simulink model "SmallScaleMicroGrid"  (R2024a)
settings: Solver=ode23tb  StartTime=0  StopTime=60*60*24  FixedStep=1/(1000)  MaxStep=50  RelTol=1e-4
PreLoadFcn:
  | load('SmallScaleMicroGridSolarLoadData24h.mat')
values from neighbouring files (symbols this model uses):
  HPD_1min = [1086.95652174 1079.71014493 1072.46376812 1065.2173913 1057.97101449 1050.72463768 1043.47826087 1036.23188406 1028.98550725 1021.73913043 1014.49275362 1007.24637681 ... (1441 elements, 1441x1)]    [SmallScaleMicroGridSolarLoadData24h.mat]
  HPT_1min = [0 60 120 180 240 300 360 420 480 540 600 660 ... (1441 elements, 1441x1)]    [SmallScaleMicroGridSolarLoadData24h.mat]
  SPD_1min = [0 0 0 0 0 0 0 0 0 0 0 0 ... (1441 elements, 1441x1)]    [SmallScaleMicroGridSolarLoadData24h.mat]
  SPT_1min = [0 60 120 180 240 300 360 420 480 540 600 660 ... (1441 elements, 1441x1)]    [SmallScaleMicroGridSolarLoadData24h.mat]
libraries: spsCurrentMeasurementLib x4, spsControlledCurrentSourceLib x3, spsSeriesRLCBranchLib x3, spsACVoltageSourceLib x1, spsGroundLib x1, spsVoltageMeasurementLib x1, spspowerguiLib x1
settings Model: ModifiedByFormat=SPS  Creator=The MathWorks, Inc.  LastModifiedBy=SPS
settings SolverCC: InitialStep=1e-4  ZeroCrossAlgorithm=Adaptive  AlgebraicLoopSolver=TrustRegion  SolverResetMethod=Robust
settings DataIOCC: SaveFormat=Array  SaveOutput=off  SaveTime=off  ReturnWorkspaceOutputs=off  SignalLoggingName=sigsOut
settings OptimizationCC: BooleanDataType=off  ExpressionDepthLimit=2147483647  InitFltsAndDblsToZero=on  LifeSpan=inf
settings DebuggingCC: AlgebraicLoopMsg=none  SaveWithParameterizedLinksMsg=none  UnderspecifiedInitializationDetection=Classic  MergeDetectMultiDrivingBlocksExec=none  SignalResolutionControl=TryResolveAllWithWarning  MultiTaskDSMMsg=warning  MultiTaskCondExecSysMsg=none  FcnCallInpInsideContextMsg=warning  UnconnectedInputMsg=warning  UnconnectedOutputMsg=warning  UnconnectedLineMsg=warning  AllowSymbolicDim=off  StateNameClashWarn=warning  SubsystemReferenceDiagnosticForUnitTest=warning  SFUnexpectedBacktrackingDiag=warning  SFNoUnconditionalDefaultTransitionDiag=warning  SFExecutionAtInitializationDiag=none  ArithmeticOperatorsInVariantConditions=warning
settings HardwareCC: ProdBitPerPointer=32  ProdBitPerSizeT=32  ProdBitPerPtrDiffT=32  ProdLargestAtomicFloat=None  ProdIntDivRoundTo=Undefined  ProdEndianess=Unspecified  ProdWordSize=32  ProdHWDeviceType=32-bit Generic  TargetUnknown=on
settings ModelReferenceCC: EnableRefExpFcnMdlSchedulingChecks=on  PropagateSignalLabelsOutOfModel=off
settings SFSimCC: SimUseLocalCustomCode=off  CustomCodeUndefinedFunction=UseInterfaceOnly
settings RTWCC: RTWUseLocalCustomCode=off  GPUComputeCapability=3.5  DLArmComputeVersion=19.05
settings CodeAppCC: StateflowObjectComments=on
settings GRTTargetCC: TargetFcnLib=ansi_tfl_tmw.mat  TargetLangStandard=C89/C90 (ANSI)  CombineOutputUpdateFcns=off  GRTInterface=on
settings ConfigComp: CovMetricSettings=dw  CovSaveCumulativeToWorkspaceVar=on  CovSaveSingleToWorkspaceVar=on  CovExternalEMLEnable=off  CovSFcnEnable=off
settings SimscapeCC: SimscapeNormalizeSystem=off

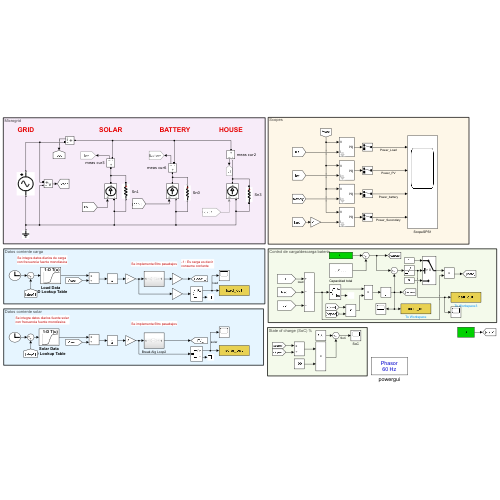
[thumbnail: Simulink's stored preview of the top-level diagram]
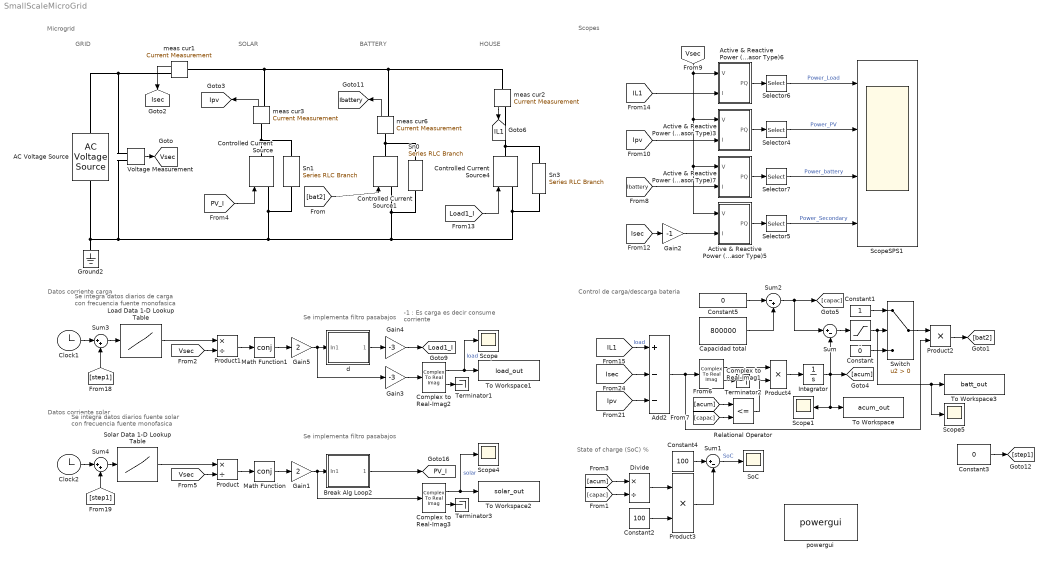
== system SmallScaleMicroGrid ==
  note: State of charge (SoC) %
  note: Control de carga/descarga bateria
  note: Microgrid
  note: Datos corriente solar
  note: Datos corriente carga
  note: SOLAR
  note: BATTERY
  note: HOUSE
  note: Se implementa filtro pasabajos
  note: Se integra datos diarios fuente solar
      | con frecuencia fuente monofasica
  note: Se integra datos diarios de carga
      | con frecuencia fuente monofasica
  note: Se implementa filtro pasabajos
  note: -1 : Es carga es decir
      | consume corriente
  note: GRID
  note: Scopes
  - : Saturate  UpperLimit=inf  LowerLimit=0
  AC Voltage Source : spsACVoltageSourceLib/AC Voltage Source  Amplitude=285  Phase=0  Frequency=60  SampleTime=0  Measurements=None  BusType=swing  Pref=10e3  Qref=0  Qmin=-inf  Qmax=+inf
  Active & Reactive Power (Phasor Type)3 : Subsystem  DialogController=POWERSYS.PowerSysDialog  mask(Active & Reactive Power (Phasor Type)){}
      mask help: Active & Reactive Power (Phasor Type)
      mask init:
      | power_initmask();
      mask Help: This block is part of a subset of blocks in the Extras library that does not have documentation associated with it, other than the block mask description.
      mask Display: disp('')
  Active & Reactive Power (Phasor Type)5 : Subsystem  DialogController=POWERSYS.PowerSysDialog  mask(Active & Reactive Power (Phasor Type)){}
      mask help: Active & Reactive Power (Phasor Type)
      mask init:
      | power_initmask();
      mask Help: This block is part of a subset of blocks in the Extras library that does not have documentation associated with it, other than the block mask description.
      mask Display: disp('')
  Active & Reactive Power (Phasor Type)6 : Subsystem  DialogController=POWERSYS.PowerSysDialog  mask(Active & Reactive Power (Phasor Type)){}
      mask help: Active & Reactive Power (Phasor Type)
      mask init:
      | power_initmask();
      mask Help: This block is part of a subset of blocks in the Extras library that does not have documentation associated with it, other than the block mask description.
      mask Display: disp('')
  Active & Reactive Power (Phasor Type)7 : Subsystem  DialogController=POWERSYS.PowerSysDialog  mask(Active & Reactive Power (Phasor Type)){}
      mask help: Active & Reactive Power (Phasor Type)
      mask init:
      | power_initmask();
      mask Help: This block is part of a subset of blocks in the Extras library that does not have documentation associated with it, other than the block mask description.
      mask Display: disp('')
  Add2 : Sum  Inputs=+--
  Break Alg Loop2 : Subsystem
  Capacidad total : Constant  Value=800000
  Clock1 : Clock
  Clock2 : Clock
  Complex to Real-Imag1 : ComplexToRealImag
  Complex to Real-Imag2 : ComplexToRealImag
  Complex to Real-Imag3 : ComplexToRealImag
  Constant : Constant  Value=0
  Constant1 : Constant
  Constant2 : Constant  Value=100
  Constant3 : Constant  Value=0
  Constant4 : Constant  Value=100
  Constant5 : Constant  Value=0
  Controlled Current Source : spsControlledCurrentSourceLib/Controlled Current Source  Initialize=on  Source_Type=AC  Amplitude=0  Phase=30  Frequency=60  Measurements=None
  Controlled Current Source1 : spsControlledCurrentSourceLib/Controlled Current Source  Initialize=on  Source_Type=AC  Amplitude=0  Phase=30  Frequency=60  Measurements=None
  Controlled Current Source4 : spsControlledCurrentSourceLib/Controlled Current Source  Initialize=on  Source_Type=AC  Amplitude=0  Phase=30  Frequency=60  Measurements=None
  Divide : Product  Inputs=*/
  Gain1 : Gain  Gain=2
  Gain2 : Gain  Gain=-1
  Gain3 : Gain  Gain=-3
  Gain4 : Gain  Gain=-3
  Gain5 : Gain  Gain=2
  Ground2 : spsGroundLib/Ground  LConnTagsString=a
  Integrator : Integrator
  Load Data 1-D Lookup Table : Lookup_n-D  NumberOfTableDimensions=1  BreakpointsForDimension1=HPT_1min  BeginIndexSearchUsingPreviousIndexResult=on  Table=HPD_1min  InternalRulePriority=Speed  RndMeth=Simplest
  Math Function : Math  Operator=conj
  Math Function1 : Math  Operator=conj
  Product : Product  Inputs=*/
  Product1 : Product  Inputs=*/
  Product2 : Product
  Product3 : Product
  Product4 : Product
  Relational Operator : RelationalOperator  Operator=<=  OutDataTypeStr=boolean  RndMeth=Simplest  InputSameDT=off
  Scope{,1,4..5} (4 alike) : Scope
  ScopeSPS1 : Scope  NumInputPorts=4
  Selector{4..7} (4 alike) : Selector  InputPortWidth=2  IndexOptions=Index vector (dialog)  Indices=1  OutputSizes=1
  Sn0 : spsSeriesRLCBranchLib/Series RLC Branch  LConnTagsString=__new0  RConnTagsString=__new0  BranchType=R  Resistance=1e6  Inductance=1e-3  SetiL0=off  InitialCurrent=0  Capacitance=1e-6  Setx0=off  InitialVoltage=0  Measurements=None
  Sn1 : spsSeriesRLCBranchLib/Series RLC Branch  LConnTagsString=__new0  RConnTagsString=__new0  BranchType=R  Resistance=1e6  Inductance=1e-3  SetiL0=off  InitialCurrent=0  Capacitance=1e-6  Setx0=off  InitialVoltage=0  Measurements=None
  Sn3 : spsSeriesRLCBranchLib/Series RLC Branch  LConnTagsString=__new0  RConnTagsString=__new0  BranchType=R  Resistance=1e6  Inductance=1e-3  SetiL0=off  InitialCurrent=0  Capacitance=1e-6  Setx0=off  InitialVoltage=0  Measurements=None
  SoC : Scope
  Solar Data 1-D Lookup Table : Lookup_n-D  NumberOfTableDimensions=1  BreakpointsForDimension1=SPT_1min  BeginIndexSearchUsingPreviousIndexResult=on  Table=SPD_1min  InternalRulePriority=Speed  RndMeth=Simplest
  Sum : Sum  Inputs=|+-
  Sum1 : Sum  Inputs=|+-
  Sum2 : Sum  Inputs=|-+
  Sum3 : Sum  Inputs=|++
  Sum4 : Sum  Inputs=|++
  Switch : Switch  Criteria=u2 > Threshold  SaturateOnIntegerOverflow=off  InputSameDT=off
  Terminator1 : Terminator
  Terminator2 : Terminator
  Terminator3 : Terminator
  To Workspace : ToWorkspace  VariableName=acum_out  SampleTime=-1
  To Workspace1 : ToWorkspace  VariableName=load_out  SampleTime=-1
  To Workspace2 : ToWorkspace  VariableName=solar_out  SampleTime=-1
  To Workspace3 : ToWorkspace  VariableName=batt_out  SampleTime=-1
  Voltage Measurement : spsVoltageMeasurementLib/Voltage Measurement  PhasorSimulation=on  OutputType=Complex  PSBequivalent=0
  d : Subsystem
  meas cur{1..3,6} (4 alike) : spsCurrentMeasurementLib/Current Measurement  PhasorSimulation=on  OutputType=Complex  PSBequivalent=0
  powergui : spspowerguiLib/powergui  SimulationMode=Phasor  SampleTime=1/60/100  frequency=60  Iterations=50  frequencyindice=60  Pbase=100e6  ErrMax=1e-4  UnitsV=kV  UnitsW=MW  buscounter=0  FunctionMessages=off  echomessages=off  EnableUseOfTLC=off  CurrentSourceSwitches=off  DisableSnubberDevices=off  DisableRonSwitches=off  DisableVfSwitches=off  DisplayEquations=off  AutomaticDiscreteSolvers=off  SolverType=Tustin  Interpol=off  ExternalGateDelay=off  methode=off  Ts=0  x0status=blocks  SPID=off  SwTol=0  HookPort=off  NonlinearTolerance=0  nMaxIteration=15  ContinueOnMaxIteration=off  RestoreLinks=warning  ResistiveCurrentMeasurement=off  Frange=[0:2:500]  Ylog=off  Xlog=on  ShowGrid=off  save=off  variable=ZData  structure=0  ZoomFFT=on  StartTime=0.0  cycles=1  DisplayStyle=1  fundamental=60  FreqAxis=off  MaxFrequency=1000  frequencyindicesteady=1  RmsSteady=1  display=off
  tag scope: IL1=global, Ibattery=global, Ipv=global, Isec=global, Load1_I=global, PV_I=global, Vsec=global
  wires:
  meas cur2/1 -> [IL1]
  meas cur1/1 -> [Isec]
  meas cur3/1 -> [Ipv]
  meas cur6/1 -> [Ibattery]
  Break Alg Loop2/1("1 ") -> [PV_I]
  Gain4/1 -> [Load1_I]
  Voltage Measurement/1 -> [Vsec]
  [Load1_I] -> Controlled Current Source4/1
  [PV_I] -> Controlled Current Source/1
  Load Data 1-D Lookup Table/1 -> Product1/1
  Product1/1 -> Math Function1/1
  Product/1 -> Math Function/1
  Solar Data 1-D Lookup Table/1 -> Product/1
  Math Function1/1 -> Gain5/1
  Gain5/1 -> Gain3/1, d/1(In1)
  Math Function/1 -> Gain1/1
  [Vsec] -> Product1/2
  [Vsec] -> Product/2
  Gain1/1 -> Complex to Real-Imag3/1, Break Alg Loop2/1(In1)
  d/1("1 ") -> Gain4/1
  [Ipv] -> Add2/3
  [Isec] -> Add2/2
  [IL1] -> Add2/1  "load"
  Add2/1 -> Product2/2, Complex to Real-Imag1/1
  [bat2] -> Controlled Current Source1/1
  Complex to Real-Imag1/2 -> Terminator2/1
  Integrator/1 -> Sum/2, [acum], Scope1/1, To Workspace/1
  Sum/1 -> -/1
  Sum2/1 -> [capac], Sum/1
  Constant/1 -> Switch/3
  -/1 -> Scope5/1, To Workspace3/1, Switch/2
  Constant1/1 -> Switch/1
  Product2/1 -> [bat2]
  Switch/1 -> Product2/1
  [acum] -> Divide/1
  [capac] -> Divide/2
  Divide/1 -> Product3/1
  Constant2/1 -> Product3/2
  [acum] -> Relational Operator/1
  [capac] -> Relational Operator/2
  Product4/1 -> Integrator/1
  Complex to Real-Imag1/1 -> Product4/1
  Relational Operator/1 -> Product4/2
  Gain2/1 -> Active & Reactive Power (Phasor Type)5/2(I)
  Active & Reactive Power (Phasor Type)6/1(PQ) -> Selector6/1
  Active & Reactive Power (Phasor Type)3/1(PQ) -> Selector4/1
  Active & Reactive Power (Phasor Type)5/1(PQ) -> Selector5/1
  [IL1] -> Active & Reactive Power (Phasor Type)6/2(I)
  [Isec] -> Gain2/1
  [Ibattery] -> Active & Reactive Power (Phasor Type)7/2(I)
  Active & Reactive Power (Phasor Type)7/1(PQ) -> Selector7/1
  [Ipv] -> Active & Reactive Power (Phasor Type)3/2(I)
  Selector4/1 -> ScopeSPS1/2  "Power_PV"
  Selector6/1 -> ScopeSPS1/1  "Power_Load"
  Selector7/1 -> ScopeSPS1/3  "Power_battery"
  Selector5/1 -> ScopeSPS1/4  "Power_Secondary"
  [Vsec] -> Active & Reactive Power (Phasor Type)3/1(V), Active & Reactive Power (Phasor Type)7/1(V), Active & Reactive Power (Phasor Type)5/1(V), Active & Reactive Power (Phasor Type)6/1(V)
  Constant4/1 -> Sum1/1
  Product3/1 -> Sum1/2
  Sum1/1 -> SoC/1  "SoC"
  Constant3/1 -> [step1]
  Clock1/1 -> Sum3/1
  Sum3/1 -> Load Data 1-D Lookup Table/1
  [step1] -> Sum3/2
  Clock2/1 -> Sum4/1
  Sum4/1 -> Solar Data 1-D Lookup Table/1
  [step1] -> Sum4/2
  Gain3/1 -> Complex to Real-Imag2/1
  Complex to Real-Imag2/1 -> Scope/1, To Workspace1/1  "load"
  Complex to Real-Imag2/2 -> Terminator1/1
  Complex to Real-Imag3/1 -> Scope4/1, To Workspace2/1  "solar"
  Complex to Real-Imag3/2 -> Terminator3/1
  Constant5/1 -> Sum2/1
  Capacidad total/1 -> Sum2/2
  connections:
  Voltage Measurement/LConn1 -- AC Voltage Source/RConn1 -- meas cur1/RConn1
  Sn1/LConn1 -- Controlled Current Source/RConn1 -- meas cur3/LConn1
  Controlled Current Source1/RConn1 -- meas cur6/LConn1 -- Sn0/LConn1
  Controlled Current Source4/LConn1 -- Controlled Current Source1/LConn1 -- Sn0/RConn1 -- Controlled Current Source/LConn1 -- Sn1/RConn1 -- Ground2/LConn1 -- AC Voltage Source/LConn1 -- Voltage Measurement/LConn2 -- Sn3/RConn1
  Controlled Current Source4/RConn1 -- meas cur2/RConn1 -- Sn3/LConn1
  meas cur1/LConn1 -- meas cur3/RConn1 -- meas cur2/LConn1 -- meas cur6/RConn1

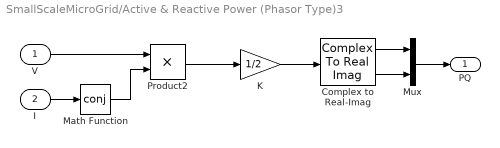
== system SmallScaleMicroGrid/Active & Reactive Power (Phasor Type)3 ==
  V : Inport
  I : Inport  Port=2
  Complex to Real-Imag : ComplexToRealImag
  K : Gain  Gain=1/2  SaturateOnIntegerOverflow=on  OutDataTypeStr=Inherit: Same as input  ParamDataTypeStr=Inherit: Same as input
  Math Function : Math  Operator=conj  SignedPower=on
  Mux : Mux  Inputs=2
  Product2 : Product  InputSameDT=on  SaturateOnIntegerOverflow=on  OutDataTypeStr=Inherit: Same as first input
  PQ : Outport  VectorParamsAs1DForOutWhenUnconnected=off
  wires:
  Mux/1 -> PQ/1
  Complex to Real-Imag/2 -> Mux/2
  Complex to Real-Imag/1 -> Mux/1
  V/1 -> Product2/1
  Math Function/1 -> Product2/2
  Product2/1 -> K/1
  K/1 -> Complex to Real-Imag/1
  I/1 -> Math Function/1

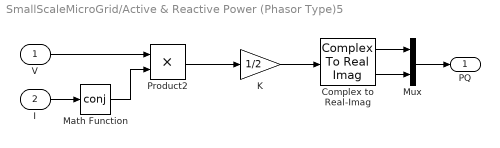
== system SmallScaleMicroGrid/Active & Reactive Power (Phasor Type)5 ==
  V : Inport
  I : Inport  Port=2
  Complex to Real-Imag : ComplexToRealImag
  K : Gain  Gain=1/2  SaturateOnIntegerOverflow=on  OutDataTypeStr=Inherit: Same as input  ParamDataTypeStr=Inherit: Same as input
  Math Function : Math  Operator=conj  SignedPower=on
  Mux : Mux  Inputs=2
  Product2 : Product  InputSameDT=on  SaturateOnIntegerOverflow=on  OutDataTypeStr=Inherit: Same as first input
  PQ : Outport  VectorParamsAs1DForOutWhenUnconnected=off
  wires:
  Mux/1 -> PQ/1
  Complex to Real-Imag/2 -> Mux/2
  Complex to Real-Imag/1 -> Mux/1
  V/1 -> Product2/1
  Math Function/1 -> Product2/2
  Product2/1 -> K/1
  K/1 -> Complex to Real-Imag/1
  I/1 -> Math Function/1

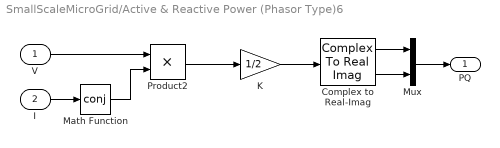
== system SmallScaleMicroGrid/Active & Reactive Power (Phasor Type)6 ==
  V : Inport
  I : Inport  Port=2
  Complex to Real-Imag : ComplexToRealImag
  K : Gain  Gain=1/2  SaturateOnIntegerOverflow=on  OutDataTypeStr=Inherit: Same as input  ParamDataTypeStr=Inherit: Same as input
  Math Function : Math  Operator=conj  SignedPower=on
  Mux : Mux  Inputs=2
  Product2 : Product  InputSameDT=on  SaturateOnIntegerOverflow=on  OutDataTypeStr=Inherit: Same as first input
  PQ : Outport  VectorParamsAs1DForOutWhenUnconnected=off
  wires:
  Mux/1 -> PQ/1
  Complex to Real-Imag/2 -> Mux/2
  Complex to Real-Imag/1 -> Mux/1
  V/1 -> Product2/1
  Math Function/1 -> Product2/2
  Product2/1 -> K/1
  K/1 -> Complex to Real-Imag/1
  I/1 -> Math Function/1

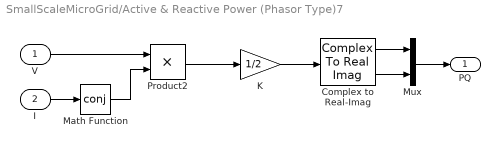
== system SmallScaleMicroGrid/Active & Reactive Power (Phasor Type)7 ==
  V : Inport
  I : Inport  Port=2
  Complex to Real-Imag : ComplexToRealImag
  K : Gain  Gain=1/2  SaturateOnIntegerOverflow=on  OutDataTypeStr=Inherit: Same as input  ParamDataTypeStr=Inherit: Same as input
  Math Function : Math  Operator=conj  SignedPower=on
  Mux : Mux  Inputs=2
  Product2 : Product  InputSameDT=on  SaturateOnIntegerOverflow=on  OutDataTypeStr=Inherit: Same as first input
  PQ : Outport  VectorParamsAs1DForOutWhenUnconnected=off
  wires:
  Mux/1 -> PQ/1
  Complex to Real-Imag/2 -> Mux/2
  Complex to Real-Imag/1 -> Mux/1
  V/1 -> Product2/1
  Math Function/1 -> Product2/2
  Product2/1 -> K/1
  K/1 -> Complex to Real-Imag/1
  I/1 -> Math Function/1

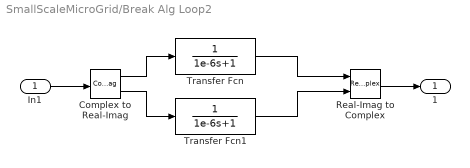
== system SmallScaleMicroGrid/Break Alg Loop2 ==
  In1 : Inport
  Complex to Real-Imag : ComplexToRealImag
  Real-Imag to Complex : RealImagToComplex
  Transfer Fcn : TransferFcn  Denominator=[1e-6 1]
  Transfer Fcn1 : TransferFcn  Denominator=[1e-6 1]
  "1 " : Outport
  wires:
  In1/1 -> Complex to Real-Imag/1
  Complex to Real-Imag/1 -> Transfer Fcn/1
  Complex to Real-Imag/2 -> Transfer Fcn1/1
  Transfer Fcn/1 -> Real-Imag to Complex/1
  Real-Imag to Complex/1 -> "1 "/1
  Transfer Fcn1/1 -> Real-Imag to Complex/2

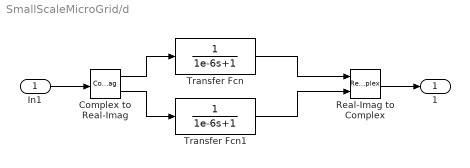
== system SmallScaleMicroGrid/d ==
  In1 : Inport
  Complex to Real-Imag : ComplexToRealImag
  Real-Imag to Complex : RealImagToComplex
  Transfer Fcn : TransferFcn  Denominator=[1e-6 1]
  Transfer Fcn1 : TransferFcn  Denominator=[1e-6 1]
  "1 " : Outport
  wires:
  Transfer Fcn1/1 -> Real-Imag to Complex/2
  Real-Imag to Complex/1 -> "1 "/1
  Transfer Fcn/1 -> Real-Imag to Complex/1
  Complex to Real-Imag/2 -> Transfer Fcn1/1
  Complex to Real-Imag/1 -> Transfer Fcn/1
  In1/1 -> Complex to Real-Imag/1
